simulink model "WaveletTraj"  (Simulink 10.1)
settings: Solver=FixedStepDiscrete  StartTime=0.0  StopTime=inf  FixedStep=Ts  RelTol=1e-3
PreLoadFcn:
  | load param
undefined symbols (not defined in the file or in its folder): c_maxsz, DiscIntNeverNeededParam, Dphival_fi, f, interp_gain, interp_uplim, phival_fi, Ts, tval_fi, w
libraries: simulink x36, dspsigops x24, dspindex x16, dspswit3 x12, simulink_extras x8
(part 1 of 4)
settings Model: Creator=Carchesion  LastModifiedBy=upattacini  ParamWorkspaceSource=ReferencedWorkspace
settings SolverCC: ZeroCrossAlgorithm=Non-adaptive
settings DataIOCC: SignalLoggingSaveFormat=ModelDataLogs  SaveOutput=off  SignalLogging=off  SaveTime=off
settings OptimizationCC: DefaultParameterBehavior=Inlined  InlineInvariantSignals=on  ExpressionDepthLimit=2147483647  StateBitsets=on  DataBitsets=on  NoFixptDivByZeroProtection=on  EfficientFloat2IntCast=on  LifeSpan=1  SimCompilerOptimization=on  EfficientTunableParamExpr=on
settings DebuggingCC: SolverPrmCheckMsg=warning  ParameterPrecisionLossMsg=none  FcnCallInpInsideContextMsg=warning  StateNameClashWarn=warning
settings HardwareCC: ProdIntDivRoundTo=Zero  ProdEndianess=BigEndian  ProdWordSize=16  ProdHWDeviceType=Generic->Custom  TargetBitPerInt=16  TargetIntDivRoundTo=Zero  TargetEndianess=BigEndian  TargetWordSize=16  TargetHWDeviceType=Freescale->DSP563xx (16-bit mode)
settings SFSimCC: SimUseLocalCustomCode=on  SimParseCustomCode=off  MATLABDynamicMemAlloc=off  CustomCodeUndefinedFunction=FilterOut
settings RTWCC: Description=Real-Time Workshop Embedded Coder (no auto configuration)  SystemTargetFile=ert.tlc  GenCodeOnly=on  GenerateMakefile=off  TemplateMakefile=ert_default_tmf  GenerateReport=on  RTWUseLocalCustomCode=on  IncludeHyperlinkInReport=on  LaunchReport=on  PortableWordSizes=on  CreateSILPILBlock=SIL  GenerateTraceInfo=on  RTWCompilerOptimization=on
settings RTWCC: CustomHeaderCode=|
  | /* Fractional Length Enxx*/
  | #define TRAJECTORY_FRACTLEN 12
  | 
  | /* Input Data Types */
  | // trigger = boolean
  | // abort = boolean
  | // mode =uint8
  | // int_mode = uint8
  | // Res = ufix32_Enxx
  | // x0 = sfix32_Enxx
  | // xf = sfix32_Enxx
  | // T = ufix16_En7
  | // c = sfix16_En7
  | // x_lim = sfix32_Enxx
  | // Ix_lim = sfix32_Enxx
  | // Dx_lim = sfix32_Enxx
  | 
  | /* Output Data Types */
  | // run = boolean
  | // x = sfix32_Enxx
  | // x_interp = sfix32_Enxx
  | // Ix = sfix32_Enxx
  | 
  | /* Modes for state x */
  | #define TRAJECTORY_MODE_NORM 0
  | #define TRAJECTORY_MODE_MJ 1
  | #define TRAJECTORY_MODE_VEL 2
  | 
  | /* Modes for integral of x */
  | #define TRAJECTORY_INT_MODE_OFF 0
  | #define TRAJECTORY_INT_MODE_NORM 1
  | #define TRAJECTORY_INT_MODE_INTERP 2
settings CodeAppCC: ForceParamTrailComments=on  IgnoreCustomStorageClasses=off  SimulinkDataObjDesc=on  CustomSymbolStrType=$R$N$M  CustomSymbolStrFcn=$N$M$F  CustomSymbolStrMacro=$N$M  InsertBlockDesc=on  InternalIdentifier=Classic
settings ERTTargetCC: GenerateSampleERTMain=on  IncludeMdlTerminateFcn=off  SuppressErrorStatus=on  PurelyIntegerCode=on  SupportNonFinite=off  SupportComplex=off  InlinedParameterPlacement=NonHierarchical  ERTCustomFileTemplate=example_file_process.tlc  GlobalDataDefinition=InSourceFile  GlobalDataReference=InSourceFile  ConvertIfToSwitch=off  SuppressUnreachableDefaultCases=off
settings ConfigComp: CovExternalEMLEnable=on

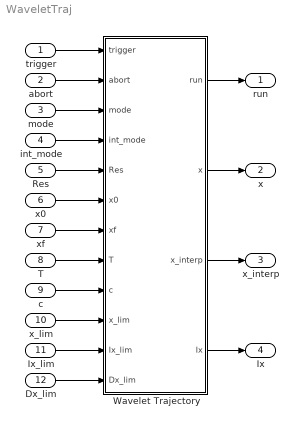
== system WaveletTraj ==
  trigger : Inport  OutDataTypeStr=boolean  PortDimensions=4
  abort : Inport  Port=2  OutDataTypeStr=boolean  PortDimensions=4
  mode : Inport  Port=3  OutDataTypeStr=uint8  PortDimensions=4
  int_mode : Inport  Port=4  OutDataTypeStr=uint8  PortDimensions=4
  Res : Inport  Port=5  OutDataTypeStr=fixdt(0,w,f)  PortDimensions=4
  x0 : Inport  Port=6  OutDataTypeStr=fixdt(1,w,f)  PortDimensions=4
  xf : Inport  Port=7  OutDataTypeStr=fixdt(1,w,f)  PortDimensions=4
  T : Inport  Port=8  OutDataTypeStr=fixdt(0,16,7)  PortDimensions=4
  c : Inport  Port=9  OutDataTypeStr=fixdt(1,16,7)  PortDimensions=[4 c_maxsz]
  x_lim : Inport  Port=10  OutDataTypeStr=fixdt(1,w,f)  PortDimensions=[4 2]
  Ix_lim : Inport  Port=11  OutDataTypeStr=fixdt(1,w,f)  PortDimensions=[4 2]
  Dx_lim : Inport  Port=12  OutDataTypeStr=fixdt(1,w,f)  PortDimensions=[4 2]
  Wavelet Trajectory : Subsystem
  run : Outport  PortDimensions=4
  x : Outport  Port=2  PortDimensions=4
  x_interp : Outport  Port=3  PortDimensions=4
  Ix : Outport  Port=4  PortDimensions=4
  wires:
  trigger/1 -> Wavelet Trajectory/1(trigger)
  Res/1 -> Wavelet Trajectory/5(Res)
  x0/1 -> Wavelet Trajectory/6(x0)
  T/1 -> Wavelet Trajectory/8(T)
  c/1 -> Wavelet Trajectory/9(c)
  Wavelet Trajectory/1(run) -> run/1
  Wavelet Trajectory/2(x) -> x/1
  Wavelet Trajectory/3(x_interp) -> x_interp/1
  xf/1 -> Wavelet Trajectory/7(xf)
  mode/1 -> Wavelet Trajectory/3(mode)
  abort/1 -> Wavelet Trajectory/2(abort)
  x_lim/1 -> Wavelet Trajectory/10(x_lim)
  Ix_lim/1 -> Wavelet Trajectory/11(Ix_lim)
  Wavelet Trajectory/4(Ix) -> Ix/1
  int_mode/1 -> Wavelet Trajectory/4(int_mode)
  Dx_lim/1 -> Wavelet Trajectory/12(Dx_lim)

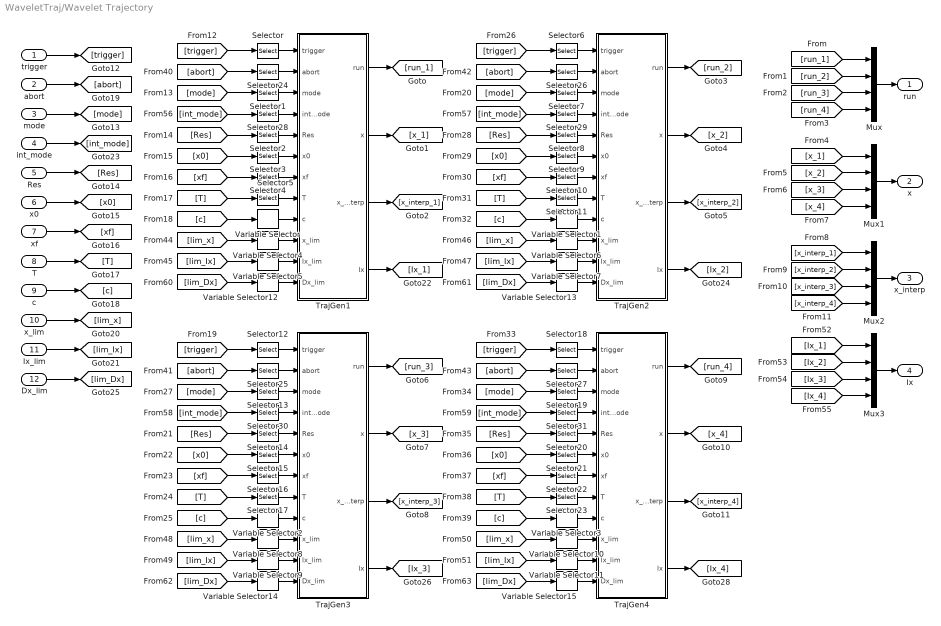
== system WaveletTraj/Wavelet Trajectory ==
  trigger : Inport
  abort : Inport  Port=2
  mode : Inport  Port=3
  int_mode : Inport  Port=4
  Res : Inport  Port=5
  x0 : Inport  Port=6
  xf : Inport  Port=7
  T : Inport  Port=8
  c : Inport  Port=9
  x_lim : Inport  Port=10
  Ix_lim : Inport  Port=11
  Dx_lim : Inport  Port=12
  Mux{,1..3} (4 alike) : Mux
  Selector{,1..5,24,28} (8 alike) : Selector  InputPortWidth=4  IndexOptions=Index vector (dialog)  Indices=1  OutputSizes=1
  Selector{6..11,26,29} (8 alike) : Selector  InputPortWidth=4  IndexOptions=Index vector (dialog)  Indices=2  OutputSizes=1
  Selector{12..17,25,30} (8 alike) : Selector  InputPortWidth=4  IndexOptions=Index vector (dialog)  Indices=3  OutputSizes=1
  Selector{18..23,27,31} (8 alike) : Selector  InputPortWidth=4  IndexOptions=Index vector (dialog)  Indices=4  OutputSizes=1
  TrajGen1 : Subsystem  TreatAsAtomicUnit=on  RTWFcnName=WaveletTrajectory
      settings: RTWFcnNameOpts=User specified
  TrajGen2 : Subsystem  TreatAsAtomicUnit=on  RTWFcnName=WaveletTrajectory
      settings: RTWFcnNameOpts=User specified
  TrajGen3 : Subsystem  TreatAsAtomicUnit=on  RTWFcnName=WaveletTrajectory
      settings: RTWFcnNameOpts=User specified
  TrajGen4 : Subsystem  TreatAsAtomicUnit=on  RTWFcnName=WaveletTrajectory
      settings: RTWFcnNameOpts=User specified
  Variable Selector{,4..5,12} (4 alike) : dspindex/Variable Selector  NumInputs=1  rowsOrCols=Rows  IdxMode=Fixed  Elements=1  ZerOneIdxMode=One-based  errmode=Clip Index  FillMode=off  FillValues=0
  Variable Selector{1,6..7,13} (4 alike) : dspindex/Variable Selector  NumInputs=1  rowsOrCols=Rows  IdxMode=Fixed  Elements=2  ZerOneIdxMode=One-based  errmode=Clip Index  FillMode=off  FillValues=0
  Variable Selector{3,10..11,15} (4 alike) : dspindex/Variable Selector  NumInputs=1  rowsOrCols=Rows  IdxMode=Fixed  Elements=4  ZerOneIdxMode=One-based  errmode=Clip Index  FillMode=off  FillValues=0
  Variable Selector{2,8..9,14} (4 alike) : dspindex/Variable Selector  NumInputs=1  rowsOrCols=Rows  IdxMode=Fixed  Elements=3  ZerOneIdxMode=One-based  errmode=Clip Index  FillMode=off  FillValues=0
  run : Outport
  x : Outport  Port=2
  x_interp : Outport  Port=3
  Ix : Outport  Port=4
  wires:
  Mux/1 -> run/1
  [run_1] -> Mux/1
  [run_2] -> Mux/2
  [run_3] -> Mux/3
  [run_4] -> Mux/4
  [x_1] -> Mux1/1
  [x_2] -> Mux1/2
  [x_3] -> Mux1/3
  [x_4] -> Mux1/4
  [x_interp_1] -> Mux2/1
  [x_interp_2] -> Mux2/2
  [x_interp_3] -> Mux2/3
  [x_interp_4] -> Mux2/4
  Mux2/1 -> x_interp/1
  Mux1/1 -> x/1
  trigger/1 -> [trigger]
  mode/1 -> [mode]
  Res/1 -> [Res]
  x0/1 -> [x0]
  xf/1 -> [xf]
  T/1 -> [T]
  c/1 -> [c]
  [trigger] -> Selector/1
  [mode] -> Selector1/1
  [Res] -> Selector2/1
  [x0] -> Selector3/1
  [xf] -> Selector4/1
  [T] -> Selector5/1
  [c] -> Variable Selector/1
  [trigger] -> Selector12/1
  [mode] -> Selector13/1
  [Res] -> Selector14/1
  [x0] -> Selector15/1
  [xf] -> Selector16/1
  [T] -> Selector17/1
  [c] -> Variable Selector2/1
  [trigger] -> Selector6/1
  [mode] -> Selector7/1
  [Res] -> Selector8/1
  [x0] -> Selector9/1
  [xf] -> Selector10/1
  [T] -> Selector11/1
  [c] -> Variable Selector1/1
  [trigger] -> Selector18/1
  [mode] -> Selector19/1
  [Res] -> Selector20/1
  [x0] -> Selector21/1
  [xf] -> Selector22/1
  [T] -> Selector23/1
  [c] -> Variable Selector3/1
  Variable Selector/1 -> TrajGen1/9(c)
  Selector5/1 -> TrajGen1/8(T)
  Selector4/1 -> TrajGen1/7(xf)
  Selector3/1 -> TrajGen1/6(x0)
  Selector2/1 -> TrajGen1/5(Res)
  Selector1/1 -> TrajGen1/3(mode)
  Selector/1 -> TrajGen1/1(trigger)
  [abort] -> Selector24/1
  Selector24/1 -> TrajGen1/2(abort)
  abort/1 -> [abort]
  TrajGen1/1(run) -> [run_1]
  TrajGen1/2(x) -> [x_1]
  TrajGen1/3(x_interp) -> [x_interp_1]
  [abort] -> Selector25/1
  [abort] -> Selector26/1
  [abort] -> Selector27/1
  Ix_lim/1 -> [lim_Ix]
  x_lim/1 -> [lim_x]
  Variable Selector4/1 -> TrajGen1/10(x_lim)
  Variable Selector5/1 -> TrajGen1/11(Ix_lim)
  [lim_x] -> Variable Selector6/1
  [lim_Ix] -> Variable Selector7/1
  [lim_x] -> Variable Selector8/1
  [lim_Ix] -> Variable Selector9/1
  [lim_x] -> Variable Selector10/1
  [lim_Ix] -> Variable Selector11/1
  TrajGen1/4(Ix) -> [Ix_1]
  [Ix_1] -> Mux3/1
  [Ix_2] -> Mux3/2
  [Ix_3] -> Mux3/3
  [Ix_4] -> Mux3/4
  Mux3/1 -> Ix/1
  [lim_x] -> Variable Selector4/1
  [lim_Ix] -> Variable Selector5/1
  int_mode/1 -> [int_mode]
  [int_mode] -> Selector28/1
  Selector28/1 -> TrajGen1/4(int_mode)
  [int_mode] -> Selector29/1
  [int_mode] -> Selector30/1
  [int_mode] -> Selector31/1
  Selector6/1 -> TrajGen2/1(trigger)
  Selector26/1 -> TrajGen2/2(abort)
  Selector7/1 -> TrajGen2/3(mode)
  Selector29/1 -> TrajGen2/4(int_mode)
  Selector8/1 -> TrajGen2/5(Res)
  Selector9/1 -> TrajGen2/6(x0)
  Selector10/1 -> TrajGen2/7(xf)
  Selector11/1 -> TrajGen2/8(T)
  Variable Selector1/1 -> TrajGen2/9(c)
  Variable Selector6/1 -> TrajGen2/10(x_lim)
  Variable Selector7/1 -> TrajGen2/11(Ix_lim)
  Selector12/1 -> TrajGen3/1(trigger)
  Selector25/1 -> TrajGen3/2(abort)
  Selector13/1 -> TrajGen3/3(mode)
  Selector30/1 -> TrajGen3/4(int_mode)
  Selector14/1 -> TrajGen3/5(Res)
  Selector15/1 -> TrajGen3/6(x0)
  Selector16/1 -> TrajGen3/7(xf)
  Selector17/1 -> TrajGen3/8(T)
  Variable Selector2/1 -> TrajGen3/9(c)
  Variable Selector8/1 -> TrajGen3/10(x_lim)
  Variable Selector9/1 -> TrajGen3/11(Ix_lim)
  Selector18/1 -> TrajGen4/1(trigger)
  Selector27/1 -> TrajGen4/2(abort)
  Selector19/1 -> TrajGen4/3(mode)
  Selector31/1 -> TrajGen4/4(int_mode)
  Selector20/1 -> TrajGen4/5(Res)
  Selector21/1 -> TrajGen4/6(x0)
  Selector22/1 -> TrajGen4/7(xf)
  Selector23/1 -> TrajGen4/8(T)
  Variable Selector3/1 -> TrajGen4/9(c)
  Variable Selector10/1 -> TrajGen4/10(x_lim)
  Variable Selector11/1 -> TrajGen4/11(Ix_lim)
  TrajGen2/1(run) -> [run_2]
  Dx_lim/1 -> [lim_Dx]
  [lim_Dx] -> Variable Selector12/1
  Variable Selector12/1 -> TrajGen1/12(Dx_lim)
  TrajGen2/2(x) -> [x_2]
  TrajGen2/3(x_interp) -> [x_interp_2]
  TrajGen2/4(Ix) -> [Ix_2]
  TrajGen3/1(run) -> [run_3]
  TrajGen3/2(x) -> [x_3]
  TrajGen3/3(x_interp) -> [x_interp_3]
  TrajGen3/4(Ix) -> [Ix_3]
  TrajGen4/1(run) -> [run_4]
  TrajGen4/2(x) -> [x_4]
  TrajGen4/3(x_interp) -> [x_interp_4]
  TrajGen4/4(Ix) -> [Ix_4]
  [lim_Dx] -> Variable Selector13/1
  Variable Selector13/1 -> TrajGen2/12(Dx_lim)
  [lim_Dx] -> Variable Selector14/1
  Variable Selector14/1 -> TrajGen3/12(Dx_lim)
  [lim_Dx] -> Variable Selector15/1
  Variable Selector15/1 -> TrajGen4/12(Dx_lim)

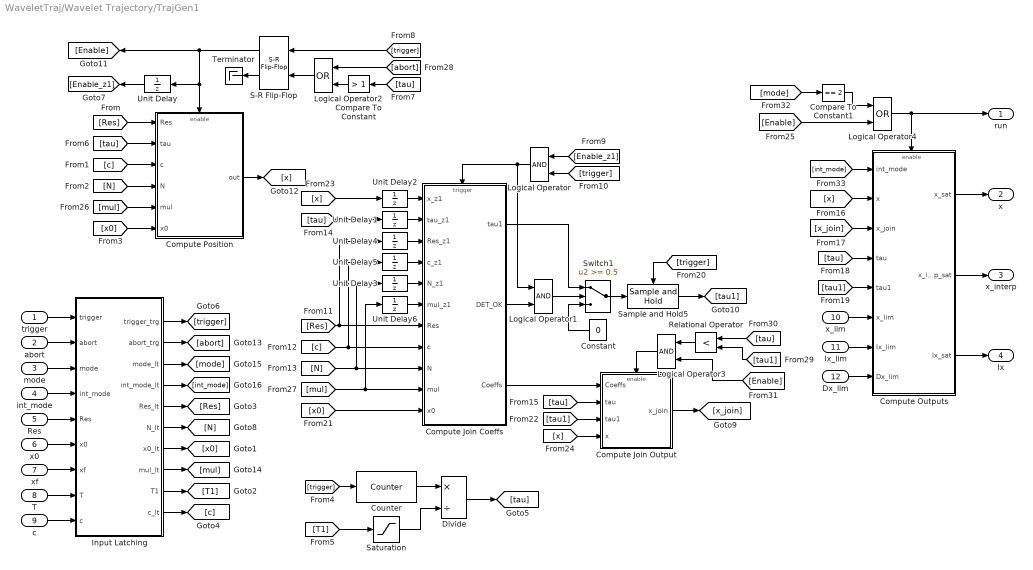
== system WaveletTraj/Wavelet Trajectory/TrajGen1 ==
  trigger : Inport  PortDimensions=1
  abort : Inport  Port=2  PortDimensions=1
  mode : Inport  Port=3  PortDimensions=1
  int_mode : Inport  Port=4  PortDimensions=1
  Res : Inport  Port=5  PortDimensions=1
  x0 : Inport  Port=6  PortDimensions=1
  xf : Inport  Port=7  PortDimensions=1
  T : Inport  Port=8  PortDimensions=1
  c : Inport  Port=9  PortDimensions=c_maxsz
  x_lim : Inport  Port=10  PortDimensions=2
  Ix_lim : Inport  Port=11  PortDimensions=2
  Dx_lim : Inport  Port=12  PortDimensions=2
  Compare To Constant : simulink/Logic and Bit Operations/Compare To Constant  SystemSampleTime=-1  relop=>  const=1  LogicOutDataTypeMode=boolean  ZeroCross=off
  Compare To Constant1 : simulink/Logic and Bit Operations/Compare To Constant  SystemSampleTime=-1  relop===  const=2  LogicOutDataTypeMode=boolean  ZeroCross=off
  Compute Join Coeffs : Subsystem  RTWFcnName=Trajectory_ComputeJoinCoeffs
      settings: RTWFcnNameOpts=User specified
  Compute Join Output : Subsystem  TreatAsAtomicUnit=on  RTWFcnName=Trajectory_ComputeJoinOutput
      settings: RTWFcnNameOpts=User specified
  Compute Outputs : Subsystem  TreatAsAtomicUnit=on  RTWFcnName=Trajectory_ComputeOutputs
      settings: RTWFcnNameOpts=User specified
  Compute Position : Subsystem  TreatAsAtomicUnit=on  RTWFcnName=Trajectory_ComputePosition
      settings: RTWFcnNameOpts=User specified
  Constant : Constant  Value=0  OutDataTypeStr=fixdt(1,w,f)
  Counter : dspswit3/Counter  Direction=Up  CountEvent=Free running  CounterSize=32 bits  MaxCount=255  InitialCount=0  Output=Count  HitValue=32  ResetInput=on  SamplesPerFrame=1  Ts=-1  CntDtype=uint32  HitDtype=Logical
  Divide : Product  Inputs=*/  OutDataTypeStr=fixdt(1,w,f)  RndMeth=Nearest  SaturateOnIntegerOverflow=on
  Input Latching : Subsystem  TreatAsAtomicUnit=on  RTWFcnName=Trajectory_InputLatching
      settings: RTWFcnNameOpts=User specified
  Logical Operator : Logic  IconShape=distinctive  AllPortsSameDT=off  OutDataTypeStr=boolean
  Logical Operator1 : Logic  IconShape=distinctive  AllPortsSameDT=off  OutDataTypeStr=boolean
  Logical Operator2 : Logic  Operator=OR  IconShape=distinctive  AllPortsSameDT=off  OutDataTypeStr=boolean
  Logical Operator3 : Logic  IconShape=distinctive  AllPortsSameDT=off  OutDataTypeStr=boolean
  Logical Operator4 : Logic  Operator=OR  IconShape=distinctive  AllPortsSameDT=off  OutDataTypeStr=boolean
  Relational Operator : RelationalOperator  Operator=<  OutDataTypeStr=boolean  RndMeth=Nearest
  S-R Flip-Flop : simulink_extras/Flip Flops/S-R Flip-Flop  SystemSampleTime=-1  initial_condition=0
  Sample and Hold5 : dspsigops/Sample and Hold  SystemSampleTime=-1  trig=Rising edge  initCond=0  latchinput=off
  Saturation : Saturate  UpperLimit=intmax('uint32')  LowerLimit=1  OutDataTypeStr=uint32  RndMeth=Nearest
  Switch1 : Switch  Threshold=0.5  OutDataTypeStr=fixdt(0,w,f)  RndMeth=Nearest  SaturateOnIntegerOverflow=on
  Terminator : Terminator
  Unit Delay{,1..6} (7 alike) : UnitDelay  SampleTime=-1
  run : Outport  PortDimensions=1
  x : Outport  Port=2  PortDimensions=1
  x_interp : Outport  Port=3  PortDimensions=1
  Ix : Outport  Port=4  PortDimensions=1
  wires:
  Unit Delay4/1 -> Compute Join Coeffs/3(Res_z1)
  [x] -> Compute Join Output/4(x)
  [tau1] -> Compute Join Output/3(tau1)
  Compute Join Output/1(x_join) -> [x_join]
  Unit Delay2/1 -> Compute Join Coeffs/1(x_z1)
  Unit Delay1/1 -> Compute Join Coeffs/2(tau_z1)
  [x0] -> Compute Position/6(x0)
  [x] -> Unit Delay2/1
  [tau] -> Unit Delay1/1
  Logical Operator1/1 -> Switch1/2
  Compute Join Coeffs/2(DET_OK) -> Logical Operator1/2
  [x0] -> Compute Join Coeffs/11(x0)
  [tau] -> Compute Join Output/2(tau)
  Compute Join Coeffs/3(Coeffs) -> Compute Join Output/1(Coeffs)
  [trigger] -> Sample and Hold5/Trigger
  Sample and Hold5/1 -> [tau1]
  Constant/1 -> Switch1/3
  Compute Join Coeffs/1(tau1) -> Switch1/1
  Switch1/1 -> Sample and Hold5/1
  Logical Operator/1 -> Logical Operator1/1, Compute Join Coeffs/Trigger
  [N] -> Compute Join Coeffs/9(N), Unit Delay3/1
  [c] -> Compute Join Coeffs/8(c), Unit Delay5/1
  [Res] -> Unit Delay4/1, Compute Join Coeffs/7(Res)
  Compute Position/1(out) -> [x]
  [trigger] -> Logical Operator/2
  [Enable_z1] -> Logical Operator/1
  [trigger] -> Counter/1
  Counter/1 -> Divide/1
  S-R Flip-Flop/1 -> Compute Position/Enable, Unit Delay/1, [Enable]
  S-R Flip-Flop/2 -> Terminator/1
  [tau] -> Compare To Constant/1
  [trigger] -> S-R Flip-Flop/1
  Saturation/1 -> Divide/2
  [tau] -> Compute Position/2(tau)
  Divide/1 -> [tau]
  [T1] -> Saturation/1
  [N] -> Compute Position/4(N)
  [c] -> Compute Position/3(c)
  [Res] -> Compute Position/1(Res)
  Unit Delay5/1 -> Compute Join Coeffs/4(c_z1)
  Unit Delay3/1 -> Compute Join Coeffs/5(N_z1)
  Unit Delay/1 -> [Enable_z1]
  trigger/1 -> Input Latching/1(trigger)
  mode/1 -> Input Latching/3(mode)
  Res/1 -> Input Latching/5(Res)
  x0/1 -> Input Latching/6(x0)
  T/1 -> Input Latching/8(T)
  c/1 -> Input Latching/9(c)
  xf/1 -> Input Latching/7(xf)
  Input Latching/1(trigger_trg) -> [trigger]
  Input Latching/5(Res_lt) -> [Res]
  Input Latching/6(N_lt) -> [N]
  Input Latching/7(x0_lt) -> [x0]
  Input Latching/9(T1) -> [T1]
  Input Latching/10(c_lt) -> [c]
  Input Latching/8(mul_lt) -> [mul]
  [mul] -> Compute Position/5(mul)
  [mul] -> Compute Join Coeffs/10(mul), Unit Delay6/1
  Unit Delay6/1 -> Compute Join Coeffs/6(mul_z1)
  abort/1 -> Input Latching/2(abort)
  Input Latching/2(abort_trg) -> [abort]
  Logical Operator2/1 -> S-R Flip-Flop/2
  [abort] -> Logical Operator2/1
  x_lim/1 -> Compute Outputs/6(x_lim)
  Ix_lim/1 -> Compute Outputs/7(Ix_lim)
  [tau1] -> Compute Outputs/5(tau1)
  [tau] -> Compute Outputs/4(tau)
  [x_join] -> Compute Outputs/3(x_join)
  [x] -> Compute Outputs/2(x)
  Compute Outputs/1(x_sat) -> x/1
  Compute Outputs/2(x_interp_sat) -> x_interp/1
  Compute Outputs/3(Ix_sat) -> Ix/1
  [tau] -> Relational Operator/1
  [tau1] -> Relational Operator/2
  Relational Operator/1 -> Logical Operator3/1
  Logical Operator3/1 -> Compute Join Output/Enable
  [Enable] -> Logical Operator3/2
  Dx_lim/1 -> Compute Outputs/8(Dx_lim)
  int_mode/1 -> Input Latching/4(int_mode)
  Input Latching/3(mode_lt) -> [mode]
  Input Latching/4(int_mode_lt) -> [int_mode]
  [int_mode] -> Compute Outputs/1(int_mode)
  [mode] -> Compare To Constant1/1
  Compare To Constant/1 -> Logical Operator2/2
  [Enable] -> Logical Operator4/2
  Logical Operator4/1 -> Compute Outputs/Enable, run/1
  Compare To Constant1/1 -> Logical Operator4/1

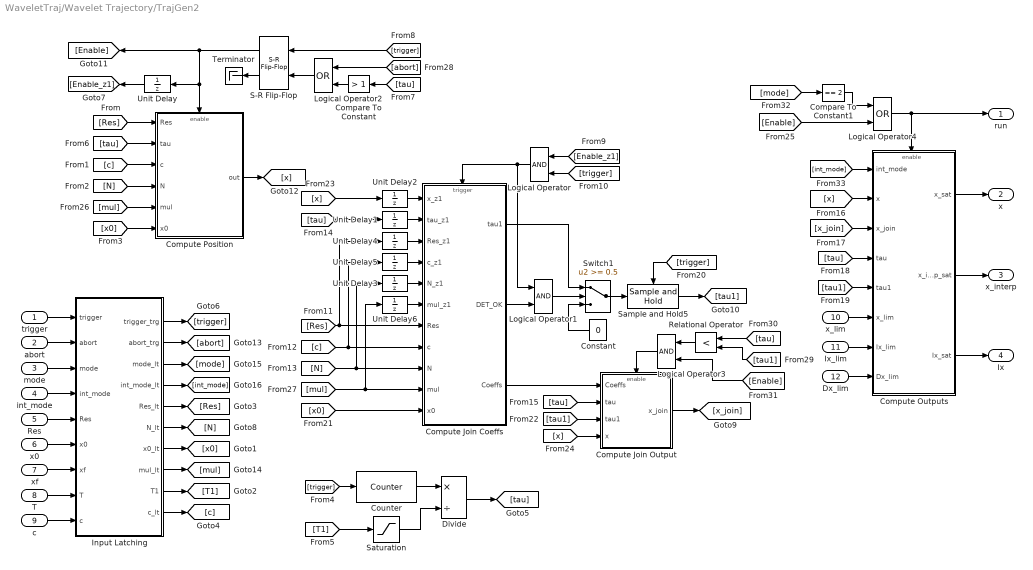
== system WaveletTraj/Wavelet Trajectory/TrajGen2 ==
  trigger : Inport  PortDimensions=1
  abort : Inport  Port=2  PortDimensions=1
  mode : Inport  Port=3  PortDimensions=1
  int_mode : Inport  Port=4  PortDimensions=1
  Res : Inport  Port=5  PortDimensions=1
  x0 : Inport  Port=6  PortDimensions=1
  xf : Inport  Port=7  PortDimensions=1
  T : Inport  Port=8  PortDimensions=1
  c : Inport  Port=9  PortDimensions=c_maxsz
  x_lim : Inport  Port=10  PortDimensions=2
  Ix_lim : Inport  Port=11  PortDimensions=2
  Dx_lim : Inport  Port=12  PortDimensions=2
  Compare To Constant : simulink/Logic and Bit Operations/Compare To Constant  SystemSampleTime=-1  relop=>  const=1  LogicOutDataTypeMode=boolean  ZeroCross=off
  Compare To Constant1 : simulink/Logic and Bit Operations/Compare To Constant  SystemSampleTime=-1  relop===  const=2  LogicOutDataTypeMode=boolean  ZeroCross=off
  Compute Join Coeffs : Subsystem  RTWFcnName=Trajectory_ComputeJoinCoeffs
      settings: RTWFcnNameOpts=User specified
  Compute Join Output : Subsystem  TreatAsAtomicUnit=on  RTWFcnName=Trajectory_ComputeJoinOutput
      settings: RTWFcnNameOpts=User specified
  Compute Outputs : Subsystem  TreatAsAtomicUnit=on  RTWFcnName=Trajectory_ComputeOutputs
      settings: RTWFcnNameOpts=User specified
  Compute Position : Subsystem  TreatAsAtomicUnit=on  RTWFcnName=Trajectory_ComputePosition
      settings: RTWFcnNameOpts=User specified
  Constant : Constant  Value=0  OutDataTypeStr=fixdt(1,w,f)
  Counter : dspswit3/Counter  Direction=Up  CountEvent=Free running  CounterSize=32 bits  MaxCount=255  InitialCount=0  Output=Count  HitValue=32  ResetInput=on  SamplesPerFrame=1  Ts=-1  CntDtype=uint32  HitDtype=Logical
  Divide : Product  Inputs=*/  OutDataTypeStr=fixdt(1,w,f)  RndMeth=Nearest  SaturateOnIntegerOverflow=on
  Input Latching : Subsystem  TreatAsAtomicUnit=on  RTWFcnName=Trajectory_InputLatching
      settings: RTWFcnNameOpts=User specified
  Logical Operator : Logic  IconShape=distinctive  AllPortsSameDT=off  OutDataTypeStr=boolean
  Logical Operator1 : Logic  IconShape=distinctive  AllPortsSameDT=off  OutDataTypeStr=boolean
  Logical Operator2 : Logic  Operator=OR  IconShape=distinctive  AllPortsSameDT=off  OutDataTypeStr=boolean
  Logical Operator3 : Logic  IconShape=distinctive  AllPortsSameDT=off  OutDataTypeStr=boolean
  Logical Operator4 : Logic  Operator=OR  IconShape=distinctive  AllPortsSameDT=off  OutDataTypeStr=boolean
  Relational Operator : RelationalOperator  Operator=<  OutDataTypeStr=boolean  RndMeth=Nearest
  S-R Flip-Flop : simulink_extras/Flip Flops/S-R Flip-Flop  SystemSampleTime=-1  initial_condition=0
  Sample and Hold5 : dspsigops/Sample and Hold  SystemSampleTime=-1  trig=Rising edge  initCond=0  latchinput=off
  Saturation : Saturate  UpperLimit=intmax('uint32')  LowerLimit=1  OutDataTypeStr=uint32  RndMeth=Nearest
  Switch1 : Switch  Threshold=0.5  OutDataTypeStr=fixdt(0,w,f)  RndMeth=Nearest  SaturateOnIntegerOverflow=on
  Terminator : Terminator
  Unit Delay{,1..6} (7 alike) : UnitDelay  SampleTime=-1
  run : Outport  PortDimensions=1
  x : Outport  Port=2  PortDimensions=1
  x_interp : Outport  Port=3  PortDimensions=1
  Ix : Outport  Port=4  PortDimensions=1
  wires:
  Compare To Constant1/1 -> Logical Operator4/1
  Logical Operator4/1 -> run/1, Compute Outputs/Enable
  [Enable] -> Logical Operator4/2
  Compare To Constant/1 -> Logical Operator2/2
  [mode] -> Compare To Constant1/1
  [int_mode] -> Compute Outputs/1(int_mode)
  Input Latching/4(int_mode_lt) -> [int_mode]
  Input Latching/3(mode_lt) -> [mode]
  int_mode/1 -> Input Latching/4(int_mode)
  Dx_lim/1 -> Compute Outputs/8(Dx_lim)
  [Enable] -> Logical Operator3/2
  Logical Operator3/1 -> Compute Join Output/Enable
  Relational Operator/1 -> Logical Operator3/1
  [tau1] -> Relational Operator/2
  [tau] -> Relational Operator/1
  Compute Outputs/3(Ix_sat) -> Ix/1
  Compute Outputs/2(x_interp_sat) -> x_interp/1
  Compute Outputs/1(x_sat) -> x/1
  [x] -> Compute Outputs/2(x)
  [x_join] -> Compute Outputs/3(x_join)
  [tau] -> Compute Outputs/4(tau)
  [tau1] -> Compute Outputs/5(tau1)
  Ix_lim/1 -> Compute Outputs/7(Ix_lim)
  x_lim/1 -> Compute Outputs/6(x_lim)
  [abort] -> Logical Operator2/1
  Logical Operator2/1 -> S-R Flip-Flop/2
  Input Latching/2(abort_trg) -> [abort]
  abort/1 -> Input Latching/2(abort)
  Unit Delay6/1 -> Compute Join Coeffs/6(mul_z1)
  [mul] -> Unit Delay6/1, Compute Join Coeffs/10(mul)
  [mul] -> Compute Position/5(mul)
  Input Latching/8(mul_lt) -> [mul]
  Input Latching/10(c_lt) -> [c]
  Input Latching/9(T1) -> [T1]
  Input Latching/7(x0_lt) -> [x0]
  Input Latching/6(N_lt) -> [N]
  Input Latching/5(Res_lt) -> [Res]
  Input Latching/1(trigger_trg) -> [trigger]
  xf/1 -> Input Latching/7(xf)
  c/1 -> Input Latching/9(c)
  T/1 -> Input Latching/8(T)
  x0/1 -> Input Latching/6(x0)
  Res/1 -> Input Latching/5(Res)
  mode/1 -> Input Latching/3(mode)
  trigger/1 -> Input Latching/1(trigger)
  Unit Delay/1 -> [Enable_z1]
  Unit Delay3/1 -> Compute Join Coeffs/5(N_z1)
  Unit Delay5/1 -> Compute Join Coeffs/4(c_z1)
  [Res] -> Compute Position/1(Res)
  [c] -> Compute Position/3(c)
  [N] -> Compute Position/4(N)
  [T1] -> Saturation/1
  Divide/1 -> [tau]
  [tau] -> Compute Position/2(tau)
  Saturation/1 -> Divide/2
  [trigger] -> S-R Flip-Flop/1
  [tau] -> Compare To Constant/1
  S-R Flip-Flop/2 -> Terminator/1
  S-R Flip-Flop/1 -> [Enable], Unit Delay/1, Compute Position/Enable
  Counter/1 -> Divide/1
  [trigger] -> Counter/1
  [Enable_z1] -> Logical Operator/1
  [trigger] -> Logical Operator/2
  Compute Position/1(out) -> [x]
  [Res] -> Compute Join Coeffs/7(Res), Unit Delay4/1
  [c] -> Unit Delay5/1, Compute Join Coeffs/8(c)
  [N] -> Unit Delay3/1, Compute Join Coeffs/9(N)
  Logical Operator/1 -> Compute Join Coeffs/Trigger, Logical Operator1/1
  Switch1/1 -> Sample and Hold5/1
  Compute Join Coeffs/1(tau1) -> Switch1/1
  Constant/1 -> Switch1/3
  Sample and Hold5/1 -> [tau1]
  [trigger] -> Sample and Hold5/Trigger
  Compute Join Coeffs/3(Coeffs) -> Compute Join Output/1(Coeffs)
  [tau] -> Compute Join Output/2(tau)
  [x0] -> Compute Join Coeffs/11(x0)
  Compute Join Coeffs/2(DET_OK) -> Logical Operator1/2
  Logical Operator1/1 -> Switch1/2
  [tau] -> Unit Delay1/1
  [x] -> Unit Delay2/1
  [x0] -> Compute Position/6(x0)
  Unit Delay1/1 -> Compute Join Coeffs/2(tau_z1)
  Unit Delay2/1 -> Compute Join Coeffs/1(x_z1)
  Compute Join Output/1(x_join) -> [x_join]
  [tau1] -> Compute Join Output/3(tau1)
  [x] -> Compute Join Output/4(x)
  Unit Delay4/1 -> Compute Join Coeffs/3(Res_z1)

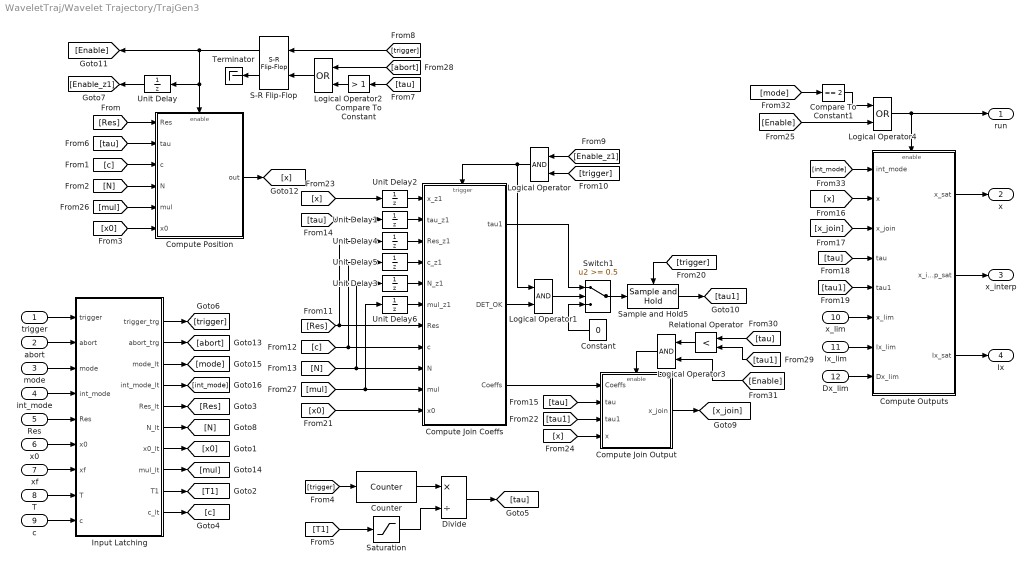
== system WaveletTraj/Wavelet Trajectory/TrajGen3 ==
  trigger : Inport  PortDimensions=1
  abort : Inport  Port=2  PortDimensions=1
  mode : Inport  Port=3  PortDimensions=1
  int_mode : Inport  Port=4  PortDimensions=1
  Res : Inport  Port=5  PortDimensions=1
  x0 : Inport  Port=6  PortDimensions=1
  xf : Inport  Port=7  PortDimensions=1
  T : Inport  Port=8  PortDimensions=1
  c : Inport  Port=9  PortDimensions=c_maxsz
  x_lim : Inport  Port=10  PortDimensions=2
  Ix_lim : Inport  Port=11  PortDimensions=2
  Dx_lim : Inport  Port=12  PortDimensions=2
  Compare To Constant : simulink/Logic and Bit Operations/Compare To Constant  SystemSampleTime=-1  relop=>  const=1  LogicOutDataTypeMode=boolean  ZeroCross=off
  Compare To Constant1 : simulink/Logic and Bit Operations/Compare To Constant  SystemSampleTime=-1  relop===  const=2  LogicOutDataTypeMode=boolean  ZeroCross=off
  Compute Join Coeffs : Subsystem  RTWFcnName=Trajectory_ComputeJoinCoeffs
      settings: RTWFcnNameOpts=User specified
  Compute Join Output : Subsystem  TreatAsAtomicUnit=on  RTWFcnName=Trajectory_ComputeJoinOutput
      settings: RTWFcnNameOpts=User specified
  Compute Outputs : Subsystem  TreatAsAtomicUnit=on  RTWFcnName=Trajectory_ComputeOutputs
      settings: RTWFcnNameOpts=User specified
  Compute Position : Subsystem  TreatAsAtomicUnit=on  RTWFcnName=Trajectory_ComputePosition
      settings: RTWFcnNameOpts=User specified
  Constant : Constant  Value=0  OutDataTypeStr=fixdt(1,w,f)
  Counter : dspswit3/Counter  Direction=Up  CountEvent=Free running  CounterSize=32 bits  MaxCount=255  InitialCount=0  Output=Count  HitValue=32  ResetInput=on  SamplesPerFrame=1  Ts=-1  CntDtype=uint32  HitDtype=Logical
  Divide : Product  Inputs=*/  OutDataTypeStr=fixdt(1,w,f)  RndMeth=Nearest  SaturateOnIntegerOverflow=on
  Input Latching : Subsystem  TreatAsAtomicUnit=on  RTWFcnName=Trajectory_InputLatching
      settings: RTWFcnNameOpts=User specified
  Logical Operator : Logic  IconShape=distinctive  AllPortsSameDT=off  OutDataTypeStr=boolean
  Logical Operator1 : Logic  IconShape=distinctive  AllPortsSameDT=off  OutDataTypeStr=boolean
  Logical Operator2 : Logic  Operator=OR  IconShape=distinctive  AllPortsSameDT=off  OutDataTypeStr=boolean
  Logical Operator3 : Logic  IconShape=distinctive  AllPortsSameDT=off  OutDataTypeStr=boolean
  Logical Operator4 : Logic  Operator=OR  IconShape=distinctive  AllPortsSameDT=off  OutDataTypeStr=boolean
  Relational Operator : RelationalOperator  Operator=<  OutDataTypeStr=boolean  RndMeth=Nearest
  S-R Flip-Flop : simulink_extras/Flip Flops/S-R Flip-Flop  SystemSampleTime=-1  initial_condition=0
  Sample and Hold5 : dspsigops/Sample and Hold  SystemSampleTime=-1  trig=Rising edge  initCond=0  latchinput=off
  Saturation : Saturate  UpperLimit=intmax('uint32')  LowerLimit=1  OutDataTypeStr=uint32  RndMeth=Nearest
  Switch1 : Switch  Threshold=0.5  OutDataTypeStr=fixdt(0,w,f)  RndMeth=Nearest  SaturateOnIntegerOverflow=on
  Terminator : Terminator
  Unit Delay{,1..6} (7 alike) : UnitDelay  SampleTime=-1
  run : Outport  PortDimensions=1
  x : Outport  Port=2  PortDimensions=1
  x_interp : Outport  Port=3  PortDimensions=1
  Ix : Outport  Port=4  PortDimensions=1
  wires:
  Unit Delay4/1 -> Compute Join Coeffs/3(Res_z1)
  [x] -> Compute Join Output/4(x)
  [tau1] -> Compute Join Output/3(tau1)
  Compute Join Output/1(x_join) -> [x_join]
  Unit Delay2/1 -> Compute Join Coeffs/1(x_z1)
  Unit Delay1/1 -> Compute Join Coeffs/2(tau_z1)
  [x0] -> Compute Position/6(x0)
  [x] -> Unit Delay2/1
  [tau] -> Unit Delay1/1
  Logical Operator1/1 -> Switch1/2
  Compute Join Coeffs/2(DET_OK) -> Logical Operator1/2
  [x0] -> Compute Join Coeffs/11(x0)
  [tau] -> Compute Join Output/2(tau)
  Compute Join Coeffs/3(Coeffs) -> Compute Join Output/1(Coeffs)
  [trigger] -> Sample and Hold5/Trigger
  Sample and Hold5/1 -> [tau1]
  Constant/1 -> Switch1/3
  Compute Join Coeffs/1(tau1) -> Switch1/1
  Switch1/1 -> Sample and Hold5/1
  Logical Operator/1 -> Logical Operator1/1, Compute Join Coeffs/Trigger
  [N] -> Compute Join Coeffs/9(N), Unit Delay3/1
  [c] -> Compute Join Coeffs/8(c), Unit Delay5/1
  [Res] -> Unit Delay4/1, Compute Join Coeffs/7(Res)
  Compute Position/1(out) -> [x]
  [trigger] -> Logical Operator/2
  [Enable_z1] -> Logical Operator/1
  [trigger] -> Counter/1
  Counter/1 -> Divide/1
  S-R Flip-Flop/1 -> Compute Position/Enable, Unit Delay/1, [Enable]
  S-R Flip-Flop/2 -> Terminator/1
  [tau] -> Compare To Constant/1
  [trigger] -> S-R Flip-Flop/1
  Saturation/1 -> Divide/2
  [tau] -> Compute Position/2(tau)
  Divide/1 -> [tau]
  [T1] -> Saturation/1
  [N] -> Compute Position/4(N)
  [c] -> Compute Position/3(c)
  [Res] -> Compute Position/1(Res)
  Unit Delay5/1 -> Compute Join Coeffs/4(c_z1)
  Unit Delay3/1 -> Compute Join Coeffs/5(N_z1)
  Unit Delay/1 -> [Enable_z1]
  trigger/1 -> Input Latching/1(trigger)
  mode/1 -> Input Latching/3(mode)
  Res/1 -> Input Latching/5(Res)
  x0/1 -> Input Latching/6(x0)
  T/1 -> Input Latching/8(T)
  c/1 -> Input Latching/9(c)
  xf/1 -> Input Latching/7(xf)
  Input Latching/1(trigger_trg) -> [trigger]
  Input Latching/5(Res_lt) -> [Res]
  Input Latching/6(N_lt) -> [N]
  Input Latching/7(x0_lt) -> [x0]
  Input Latching/9(T1) -> [T1]
  Input Latching/10(c_lt) -> [c]
  Input Latching/8(mul_lt) -> [mul]
  [mul] -> Compute Position/5(mul)
  [mul] -> Compute Join Coeffs/10(mul), Unit Delay6/1
  Unit Delay6/1 -> Compute Join Coeffs/6(mul_z1)
  abort/1 -> Input Latching/2(abort)
  Input Latching/2(abort_trg) -> [abort]
  Logical Operator2/1 -> S-R Flip-Flop/2
  [abort] -> Logical Operator2/1
  x_lim/1 -> Compute Outputs/6(x_lim)
  Ix_lim/1 -> Compute Outputs/7(Ix_lim)
  [tau1] -> Compute Outputs/5(tau1)
  [tau] -> Compute Outputs/4(tau)
  [x_join] -> Compute Outputs/3(x_join)
  [x] -> Compute Outputs/2(x)
  Compute Outputs/1(x_sat) -> x/1
  Compute Outputs/2(x_interp_sat) -> x_interp/1
  Compute Outputs/3(Ix_sat) -> Ix/1
  [tau] -> Relational Operator/1
  [tau1] -> Relational Operator/2
  Relational Operator/1 -> Logical Operator3/1
  Logical Operator3/1 -> Compute Join Output/Enable
  [Enable] -> Logical Operator3/2
  Dx_lim/1 -> Compute Outputs/8(Dx_lim)
  int_mode/1 -> Input Latching/4(int_mode)
  Input Latching/3(mode_lt) -> [mode]
  Input Latching/4(int_mode_lt) -> [int_mode]
  [int_mode] -> Compute Outputs/1(int_mode)
  [mode] -> Compare To Constant1/1
  Compare To Constant/1 -> Logical Operator2/2
  [Enable] -> Logical Operator4/2
  Logical Operator4/1 -> Compute Outputs/Enable, run/1
  Compare To Constant1/1 -> Logical Operator4/1

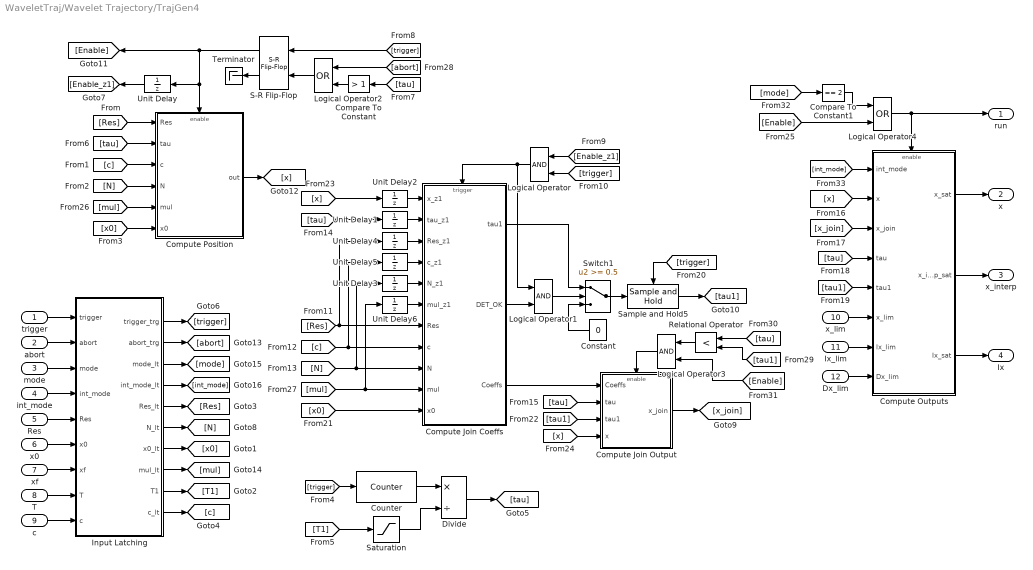
== system WaveletTraj/Wavelet Trajectory/TrajGen4 ==
  trigger : Inport  PortDimensions=1
  abort : Inport  Port=2  PortDimensions=1
  mode : Inport  Port=3  PortDimensions=1
  int_mode : Inport  Port=4  PortDimensions=1
  Res : Inport  Port=5  PortDimensions=1
  x0 : Inport  Port=6  PortDimensions=1
  xf : Inport  Port=7  PortDimensions=1
  T : Inport  Port=8  PortDimensions=1
  c : Inport  Port=9  PortDimensions=c_maxsz
  x_lim : Inport  Port=10  PortDimensions=2
  Ix_lim : Inport  Port=11  PortDimensions=2
  Dx_lim : Inport  Port=12  PortDimensions=2
  Compare To Constant : simulink/Logic and Bit Operations/Compare To Constant  SystemSampleTime=-1  relop=>  const=1  LogicOutDataTypeMode=boolean  ZeroCross=off
  Compare To Constant1 : simulink/Logic and Bit Operations/Compare To Constant  SystemSampleTime=-1  relop===  const=2  LogicOutDataTypeMode=boolean  ZeroCross=off
  Compute Join Coeffs : Subsystem  RTWFcnName=Trajectory_ComputeJoinCoeffs
      settings: RTWFcnNameOpts=User specified
  Compute Join Output : Subsystem  TreatAsAtomicUnit=on  RTWFcnName=Trajectory_ComputeJoinOutput
      settings: RTWFcnNameOpts=User specified
  Compute Outputs : Subsystem  TreatAsAtomicUnit=on  RTWFcnName=Trajectory_ComputeOutputs
      settings: RTWFcnNameOpts=User specified
  Compute Position : Subsystem  TreatAsAtomicUnit=on  RTWFcnName=Trajectory_ComputePosition
      settings: RTWFcnNameOpts=User specified
  Constant : Constant  Value=0  OutDataTypeStr=fixdt(1,w,f)
  Counter : dspswit3/Counter  Direction=Up  CountEvent=Free running  CounterSize=32 bits  MaxCount=255  InitialCount=0  Output=Count  HitValue=32  ResetInput=on  SamplesPerFrame=1  Ts=-1  CntDtype=uint32  HitDtype=Logical
  Divide : Product  Inputs=*/  OutDataTypeStr=fixdt(1,w,f)  RndMeth=Nearest  SaturateOnIntegerOverflow=on
  Input Latching : Subsystem  TreatAsAtomicUnit=on  RTWFcnName=Trajectory_InputLatching
      settings: RTWFcnNameOpts=User specified
  Logical Operator : Logic  IconShape=distinctive  AllPortsSameDT=off  OutDataTypeStr=boolean
  Logical Operator1 : Logic  IconShape=distinctive  AllPortsSameDT=off  OutDataTypeStr=boolean
  Logical Operator2 : Logic  Operator=OR  IconShape=distinctive  AllPortsSameDT=off  OutDataTypeStr=boolean
  Logical Operator3 : Logic  IconShape=distinctive  AllPortsSameDT=off  OutDataTypeStr=boolean
  Logical Operator4 : Logic  Operator=OR  IconShape=distinctive  AllPortsSameDT=off  OutDataTypeStr=boolean
  Relational Operator : RelationalOperator  Operator=<  OutDataTypeStr=boolean  RndMeth=Nearest
  S-R Flip-Flop : simulink_extras/Flip Flops/S-R Flip-Flop  SystemSampleTime=-1  initial_condition=0
  Sample and Hold5 : dspsigops/Sample and Hold  SystemSampleTime=-1  trig=Rising edge  initCond=0  latchinput=off
  Saturation : Saturate  UpperLimit=intmax('uint32')  LowerLimit=1  OutDataTypeStr=uint32  RndMeth=Nearest
  Switch1 : Switch  Threshold=0.5  OutDataTypeStr=fixdt(0,w,f)  RndMeth=Nearest  SaturateOnIntegerOverflow=on
  Terminator : Terminator
  Unit Delay{,1..6} (7 alike) : UnitDelay  SampleTime=-1
  run : Outport  PortDimensions=1
  x : Outport  Port=2  PortDimensions=1
  x_interp : Outport  Port=3  PortDimensions=1
  Ix : Outport  Port=4  PortDimensions=1
  wires:
  Compare To Constant1/1 -> Logical Operator4/1
  Logical Operator4/1 -> run/1, Compute Outputs/Enable
  [Enable] -> Logical Operator4/2
  Compare To Constant/1 -> Logical Operator2/2
  [mode] -> Compare To Constant1/1
  [int_mode] -> Compute Outputs/1(int_mode)
  Input Latching/4(int_mode_lt) -> [int_mode]
  Input Latching/3(mode_lt) -> [mode]
  int_mode/1 -> Input Latching/4(int_mode)
  Dx_lim/1 -> Compute Outputs/8(Dx_lim)
  [Enable] -> Logical Operator3/2
  Logical Operator3/1 -> Compute Join Output/Enable
  Relational Operator/1 -> Logical Operator3/1
  [tau1] -> Relational Operator/2
  [tau] -> Relational Operator/1
  Compute Outputs/3(Ix_sat) -> Ix/1
  Compute Outputs/2(x_interp_sat) -> x_interp/1
  Compute Outputs/1(x_sat) -> x/1
  [x] -> Compute Outputs/2(x)
  [x_join] -> Compute Outputs/3(x_join)
  [tau] -> Compute Outputs/4(tau)
  [tau1] -> Compute Outputs/5(tau1)
  Ix_lim/1 -> Compute Outputs/7(Ix_lim)
  x_lim/1 -> Compute Outputs/6(x_lim)
  [abort] -> Logical Operator2/1
  Logical Operator2/1 -> S-R Flip-Flop/2
  Input Latching/2(abort_trg) -> [abort]
  abort/1 -> Input Latching/2(abort)
  Unit Delay6/1 -> Compute Join Coeffs/6(mul_z1)
  [mul] -> Unit Delay6/1, Compute Join Coeffs/10(mul)
  [mul] -> Compute Position/5(mul)
  Input Latching/8(mul_lt) -> [mul]
  Input Latching/10(c_lt) -> [c]
  Input Latching/9(T1) -> [T1]
  Input Latching/7(x0_lt) -> [x0]
  Input Latching/6(N_lt) -> [N]
  Input Latching/5(Res_lt) -> [Res]
  Input Latching/1(trigger_trg) -> [trigger]
  xf/1 -> Input Latching/7(xf)
  c/1 -> Input Latching/9(c)
  T/1 -> Input Latching/8(T)
  x0/1 -> Input Latching/6(x0)
  Res/1 -> Input Latching/5(Res)
  mode/1 -> Input Latching/3(mode)
  trigger/1 -> Input Latching/1(trigger)
  Unit Delay/1 -> [Enable_z1]
  Unit Delay3/1 -> Compute Join Coeffs/5(N_z1)
  Unit Delay5/1 -> Compute Join Coeffs/4(c_z1)
  [Res] -> Compute Position/1(Res)
  [c] -> Compute Position/3(c)
  [N] -> Compute Position/4(N)
  [T1] -> Saturation/1
  Divide/1 -> [tau]
  [tau] -> Compute Position/2(tau)
  Saturation/1 -> Divide/2
  [trigger] -> S-R Flip-Flop/1
  [tau] -> Compare To Constant/1
  S-R Flip-Flop/2 -> Terminator/1
  S-R Flip-Flop/1 -> [Enable], Unit Delay/1, Compute Position/Enable
  Counter/1 -> Divide/1
  [trigger] -> Counter/1
  [Enable_z1] -> Logical Operator/1
  [trigger] -> Logical Operator/2
  Compute Position/1(out) -> [x]
  [Res] -> Compute Join Coeffs/7(Res), Unit Delay4/1
  [c] -> Unit Delay5/1, Compute Join Coeffs/8(c)
  [N] -> Unit Delay3/1, Compute Join Coeffs/9(N)
  Logical Operator/1 -> Compute Join Coeffs/Trigger, Logical Operator1/1
  Switch1/1 -> Sample and Hold5/1
  Compute Join Coeffs/1(tau1) -> Switch1/1
  Constant/1 -> Switch1/3
  Sample and Hold5/1 -> [tau1]
  [trigger] -> Sample and Hold5/Trigger
  Compute Join Coeffs/3(Coeffs) -> Compute Join Output/1(Coeffs)
  [tau] -> Compute Join Output/2(tau)
  [x0] -> Compute Join Coeffs/11(x0)
  Compute Join Coeffs/2(DET_OK) -> Logical Operator1/2
  Logical Operator1/1 -> Switch1/2
  [tau] -> Unit Delay1/1
  [x] -> Unit Delay2/1
  [x0] -> Compute Position/6(x0)
  Unit Delay1/1 -> Compute Join Coeffs/2(tau_z1)
  Unit Delay2/1 -> Compute Join Coeffs/1(x_z1)
  Compute Join Output/1(x_join) -> [x_join]
  [tau1] -> Compute Join Output/3(tau1)
  [x] -> Compute Join Output/4(x)
  Unit Delay4/1 -> Compute Join Coeffs/3(Res_z1)

== system WaveletTraj/Wavelet Trajectory/TrajGen1/Compute Join Coeffs ==
  x_z1 : Inport
  tau_z1 : Inport  Port=2
  Res_z1 : Inport  Port=3
  c_z1 : Inport  Port=4
  N_z1 : Inport  Port=5
  mul_z1 : Inport  Port=6
  Res : Inport  Port=7
  c : Inport  Port=8
  N : Inport  Port=9
  mul : Inport  Port=10
  x0 : Inport  Port=11
  Trigger : TriggerPort  VariantControl=(inherit)  StatesWhenEnabling=reset
  Abs : Abs  RndMeth=Nearest  SaturateOnIntegerOverflow=on
  Constant : Constant  Value=0  OutDataTypeStr=fixdt(1,w,f)
  Derivative1 in tau : Subsystem  TreatAsAtomicUnit=on  RTWFcnName=Trajectory_Derivative
      settings: RTWFcnNameOpts=User specified
  Derivative2 in 0 : Subsystem  TreatAsAtomicUnit=on  RTWFcnName=Trajectory_Derivative
      settings: RTWFcnNameOpts=User specified
  Derivative2 in tau1 : Subsystem  TreatAsAtomicUnit=on  RTWFcnName=Trajectory_Derivative
      settings: RTWFcnNameOpts=User specified
  Find Coeffs : Subsystem  TreatAsAtomicUnit=on  RTWFcnName=Trajectory_FindCoeffs
      settings: RTWFcnNameOpts=User specified
  Gain : Gain  Gain=interp_gain  ParamDataTypeStr=fixdt(1,w,f)  RndMeth=Nearest  SaturateOnIntegerOverflow=on  OutDataTypeStr=Inherit: Same as input
  Position2 in tau1 : Subsystem  TreatAsAtomicUnit=on  RTWFcnName=Trajectory_Position
      settings: RTWFcnNameOpts=User specified
  Product{,1..3} (4 alike) : Product  OutDataTypeStr=fixdt(1,w,f)  RndMeth=Nearest  SaturateOnIntegerOverflow=on
  Saturation1 : Saturate  UpperLimit=interp_uplim  LowerLimit=0  OutDataTypeStr=fixdt(1,w,f)  RndMeth=Nearest
  Sum1 : Sum  Inputs=++|  OutDataTypeStr=fixdt(1,w,f)  RndMeth=Nearest  SaturateOnIntegerOverflow=on
  Sum2 : Sum  Inputs=|+-  OutDataTypeStr=fixdt(1,w,f)  RndMeth=Nearest  SaturateOnIntegerOverflow=on
  tau1 : Outport
  DET_OK : Outport  Port=2
  Coeffs : Outport  Port=3
  wires:
  N_z1/1 -> Derivative1 in tau/4(N)
  Res_z1/1 -> Derivative1 in tau/1(Res)
  Find Coeffs/1(DET_OK) -> DET_OK/1
  tau_z1/1 -> Derivative1 in tau/2(tau)
  c_z1/1 -> Derivative1 in tau/3(c)
  x0/1 -> Sum1/1
  Sum1/1 -> [out2]
  Saturation1/1 -> [tau1], tau1/1
  Find Coeffs/2(Coeffs) -> Coeffs/1
  [Dout2] -> Find Coeffs/5(Dout2)
  [out2] -> Find Coeffs/4(out2)
  [Dout1] -> Find Coeffs/3(Dout1)
  [out1] -> Find Coeffs/2(out1)
  [tau1] -> Find Coeffs/1(tau1)
  x_z1/1 -> [out1]
  [tau1] -> Derivative2 in tau1/2(tau), Position2 in tau1/2(tau)
  Gain/1 -> Saturation1/1
  Abs/1 -> Gain/1
  Sum2/1 -> Abs/1
  N/1 -> Derivative2 in 0/4(N), Derivative2 in tau1/4(N), Position2 in tau1/4(N)
  c/1 -> Derivative2 in 0/3(c), Derivative2 in tau1/3(c), Position2 in tau1/3(c)
  Constant/1 -> Derivative2 in 0/2(tau)
  Res/1 -> Derivative2 in 0/1(Res), Derivative2 in tau1/1(Res), Position2 in tau1/1(Res)
  Product/1 -> Sum1/2
  Derivative1 in tau/1(out) -> Product1/2
  Product1/1 -> Sum2/1, [Dout1]
  mul_z1/1 -> Product1/1
  Derivative2 in 0/1(out) -> Product2/2
  Product2/1 -> Sum2/2
  Derivative2 in tau1/1(out) -> Product3/2
  Product3/1 -> [Dout2]
  Position2 in tau1/1(out) -> Product/2
  mul/1 -> Product2/1, Product/1, Product3/1

== system WaveletTraj/Wavelet Trajectory/TrajGen1/Compute Join Output ==
  Coeffs : Inport
  tau : Inport  Port=2
  tau1 : Inport  Port=3
  x : Inport  Port=4
  Enable : EnablePort
  CalcPoly : Subsystem
  CalcRho : Subsystem
  Product : Product  OutDataTypeStr=fixdt(1,w,f)  RndMeth=Nearest  SaturateOnIntegerOverflow=on
  Product1 : Product  OutDataTypeStr=fixdt(1,w,f)  RndMeth=Nearest  SaturateOnIntegerOverflow=on
  Sum2 : Sum  Inputs=|++  OutDataTypeStr=fixdt(1,w,f)  RndMeth=Nearest  SaturateOnIntegerOverflow=on
  x_join : Outport
  wires:
  x/1 -> Product1/2
  CalcRho/2(Rho2) -> Product1/1
  Sum2/1 -> x_join/1
  Product1/1 -> Sum2/2
  Product/1 -> Sum2/1
  CalcRho/1(Rho1) -> Product/2
  CalcPoly/1(out_poly3) -> Product/1
  tau1/1 -> CalcRho/2(tau1)
  Coeffs/1 -> CalcPoly/2(Coeffs)
  tau/1 -> CalcRho/1(tau), CalcPoly/1(tau)

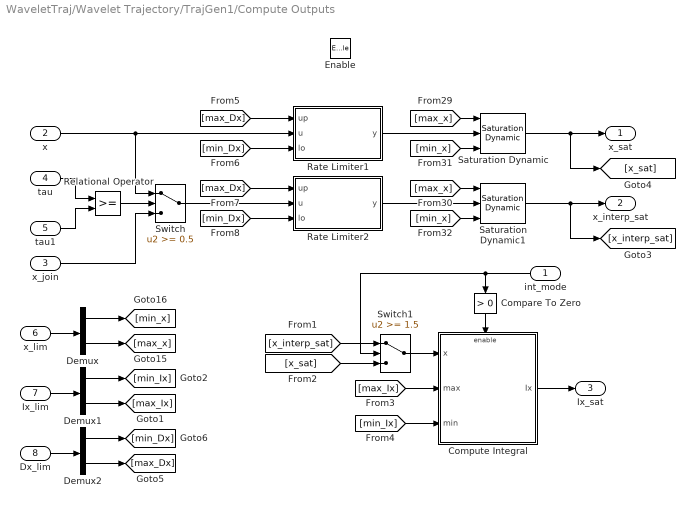
== system WaveletTraj/Wavelet Trajectory/TrajGen1/Compute Outputs ==
  int_mode : Inport
  x : Inport  Port=2
  x_join : Inport  Port=3
  tau : Inport  Port=4
  tau1 : Inport  Port=5
  x_lim : Inport  Port=6
  Ix_lim : Inport  Port=7
  Dx_lim : Inport  Port=8
  Enable : EnablePort
  Compare To Zero : simulink/Logic and Bit Operations/Compare To Zero  SystemSampleTime=-1  relop=>  LogicOutDataTypeMode=boolean  ZeroCross=off
  Compute Integral : Subsystem  TreatAsAtomicUnit=on  RTWFcnName=Trajectory_ComputeIntegral
      settings: RTWFcnNameOpts=User specified
  Demux : Demux  Outputs=2
  Demux1 : Demux  Outputs=2
  Demux2 : Demux  Outputs=2
  Rate Limiter1 : Subsystem  TreatAsAtomicUnit=on  RTWFcnName=Trajectory_RateLimiter
      settings: RTWFcnNameOpts=User specified
      mask Display:
      | disp('Rate\nLimiter');
      | port_label('input',1,'up');
      | port_label('input',2,'u');
      | port_label('input',3,'lo');
      | port_label('output',1,'y');
  Rate Limiter2 : Subsystem  TreatAsAtomicUnit=on  RTWFcnName=Trajectory_RateLimiter
      settings: RTWFcnNameOpts=User specified
      mask Display:
      | disp('Rate\nLimiter');
      | port_label('input',1,'up');
      | port_label('input',2,'u');
      | port_label('input',3,'lo');
      | port_label('output',1,'y');
  Relational Operator : RelationalOperator  OutDataTypeStr=boolean  RndMeth=Nearest
  Saturation Dynamic : simulink/Discontinuities/Saturation Dynamic  SystemSampleTime=-1  OutMin=[]  OutMax=[]  OutDataTypeStr=fixdt(1,w,f)  OutputDataTypeScalingMode=Specify via dialog  OutDataType=fixdt(1,w,f)  OutScaling=[]  RndMeth=Nearest  DoSatur=on
  Saturation Dynamic1 : simulink/Discontinuities/Saturation Dynamic  SystemSampleTime=-1  OutMin=[]  OutMax=[]  OutDataTypeStr=fixdt(1,w,f)  OutputDataTypeScalingMode=Specify via dialog  OutDataType=fixdt(1,w,f)  OutScaling=[]  RndMeth=Nearest  DoSatur=on
  Switch : Switch  Threshold=0.5  OutDataTypeStr=fixdt(1,w,f)  RndMeth=Nearest  SaturateOnIntegerOverflow=on
  Switch1 : Switch  Threshold=1.5  OutDataTypeStr=fixdt(1,w,f)  RndMeth=Nearest  SaturateOnIntegerOverflow=on
  x_sat : Outport
  x_interp_sat : Outport  Port=2
  Ix_sat : Outport  Port=3
  wires:
  x/1 -> Switch/1, Rate Limiter1/2(u)
  [min_x] -> Saturation Dynamic1/3
  [min_x] -> Saturation Dynamic/3
  [max_x] -> Saturation Dynamic1/1
  [max_x] -> Saturation Dynamic/1
  Relational Operator/1 -> Switch/2
  Saturation Dynamic/1 -> x_sat/1, [x_sat]
  tau/1 -> Relational Operator/1
  Saturation Dynamic1/1 -> x_interp_sat/1, [x_interp_sat]
  tau1/1 -> Relational Operator/2
  x_join/1 -> Switch/3
  Demux/1 -> [min_x]
  Demux/2 -> [max_x]
  Demux1/1 -> [min_Ix]
  Demux1/2 -> [max_Ix]
  [max_Ix] -> Compute Integral/2(max)
  [min_Ix] -> Compute Integral/3(min)
  Compute Integral/1(Ix) -> Ix_sat/1
  x_lim/1 -> Demux/1
  Ix_lim/1 -> Demux1/1
  [x_interp_sat] -> Switch1/1
  [x_sat] -> Switch1/3
  Switch1/1 -> Compute Integral/1(x)
  int_mode/1 -> Compare To Zero/1, Switch1/2
  Compare To Zero/1 -> Compute Integral/Enable
  Demux2/1 -> [min_Dx]
  Demux2/2 -> [max_Dx]
  Dx_lim/1 -> Demux2/1
  Rate Limiter1/1(y) -> Saturation Dynamic/2
  Rate Limiter2/1(y) -> Saturation Dynamic1/2
  Switch/1 -> Rate Limiter2/2(u)
  [max_Dx] -> Rate Limiter1/1(up)
  [min_Dx] -> Rate Limiter1/3(lo)
  [min_Dx] -> Rate Limiter2/3(lo)
  [max_Dx] -> Rate Limiter2/1(up)

== system WaveletTraj/Wavelet Trajectory/TrajGen1/Compute Position ==
  Res : Inport  PortDimensions=1
  tau : Inport  Port=2  PortDimensions=1
  c : Inport  Port=3  PortDimensions=c_maxsz
  N : Inport  Port=4  PortDimensions=1
  mul : Inport  Port=5  PortDimensions=1
  x0 : Inport  Port=6  PortDimensions=1
  Enable : EnablePort
  Position : Subsystem  TreatAsAtomicUnit=on  RTWFcnName=Trajectory_Position
      settings: RTWFcnNameOpts=User specified
  Product : Product  OutDataTypeStr=fixdt(1,w,f)  RndMeth=Nearest  SaturateOnIntegerOverflow=on
  Sum1 : Sum  Inputs=|++  OutDataTypeStr=fixdt(1,w,f)  RndMeth=Nearest  SaturateOnIntegerOverflow=on
  out : Outport  PortDimensions=1
  wires:
  x0/1 -> Sum1/2
  Sum1/1 -> out/1
  N/1 -> Position/4(N)
  c/1 -> Position/3(c)
  tau/1 -> Position/2(tau)
  Res/1 -> Position/1(Res)
  Position/1(out) -> Product/1
  Product/1 -> Sum1/1
  mul/1 -> Product/2
